simulink model "NREL5MW_FBSWE_SLOW3DOF_IPC"  (R2021b)
settings: Solver=ode4  StartTime=0.0  StopTime=Parameter.Time.TMax  FixedStep=Parameter.Time.dt  RelTol=1e-3  EnableMultiTasking=on
values from neighbouring files (symbols this model uses):
  Parameter = NREL5MWDefaultParameter_FBSWE_IPC(Parameter)    [Exercise09_IndividualPitchControllerTest.m]
undefined symbols (not defined in the file or in its folder): x2_max, x2_min, x2_t0
libraries: simulink x4
(part 2 of 2)

== matlab function NREL5MW_FBSWE_SLOW3DOF_IPC/FBSWE/Individual Pitch Controllers/ColemanTransformation ==
  data: x_0 output; x_V output; x_H output; x_1 input; x_2 input; x_3 input; psi_1 input
function [x_0,x_V,x_H] = ColemanTransformation(x_1,x_2,x_3,psi_1)

% Coleman Transformation
x_0 = 0; % Dummy
x_V = 0; % Dummy
x_H = 0; % Dummy

end

== matlab function NREL5MW_FBSWE_SLOW3DOF_IPC/FBSWE/Torque Controller/LimitsAndReferenceValueTC/LimitsAndReferenceValueTC ==
  settings: fimath=|
      | fimath(...
      | 'RoundMode', 'floor',...
      | 'OverflowMode', 'wrap',...
      | 'ProductMode', 'KeepLSB', 'ProductWordLength', 32,...
      | 'SumMode', 'KeepLSB', 'SumWordLength', 32,...
      | 'CastBeforeSum', false)
  data: Omega_g_ref output; M_g_ub output; M_g_lb output; Omega_g input; Delta_Omega_g input; Omega_g_1d5 input; k input; Omega_g_rated input; M_g_rated input; M_g_max input
function [Omega_g_ref,M_g_ub,M_g_lb] = LimitsAndReferenceValueTC(...
    Omega_g,Delta_Omega_g,...               % signals
    Omega_g_1d5,...                         % Region 1.5 parameters
    k,...                                   % Region   2 parameters
    Omega_g_rated,...                       % Region 2.5 parameters
    M_g_rated,...                           % Region   3 parameters
    M_g_max)                                % limits
 


%% Internals
Omega_g_R2Switch    = (Omega_g_1d5+Omega_g_rated)/2;

%% State Machine
if Omega_g<Omega_g_R2Switch
    Omega_g_ref             = Omega_g_1d5;
	M_g_lb                  = 0;
    M_g_ub                  = k*Omega_g^2;
else  
    if Delta_Omega_g<0
        Omega_g_ref     	= Omega_g_rated;
        M_g_lb            	= k*Omega_g^2;
        M_g_ub           	= M_g_rated;%min(M_g_rated*Omega_g_rated/Omega_g,M_g_max);
    else
        Omega_g_ref         = Omega_g_rated-Delta_Omega_g;
        M_g_lb              = k*Omega_g^2;
        M_g_ub              = M_g_rated;%min(M_g_rated*Omega_g_rated/Omega_g,M_g_max);
    end       
end

end
